simulink model "ALU1bit"  (R2024a)
settings: Solver=VariableStepAuto  StartTime=0.0  StopTime=10.0  RelTol=1e-3
settings Model: Creator=tusha  LastModifiedBy=tusha

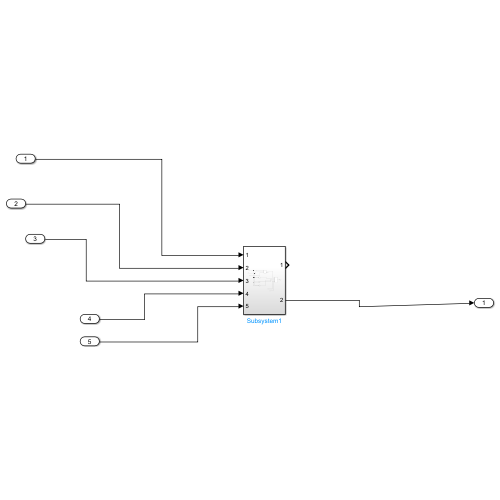
[thumbnail: Simulink's stored preview of the top-level diagram]
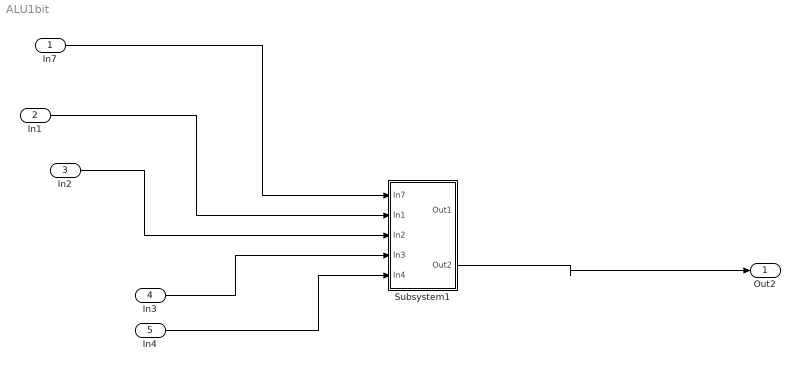
== system ALU1bit ==
  In7 : Inport
  In1 : Inport  Port=2
  In2 : Inport  Port=3
  In3 : Inport  Port=4
  In4 : Inport  Port=5
  Subsystem1 : Subsystem
  Out2 : Outport
  wires:
  In7/1 -> Subsystem1/1(In7)
  In1/1 -> Subsystem1/2(In1)
  In2/1 -> Subsystem1/3(In2)
  In3/1 -> Subsystem1/4(In3)
  In4/1 -> Subsystem1/5(In4)
  Subsystem1/2(Out2) -> Out2/1

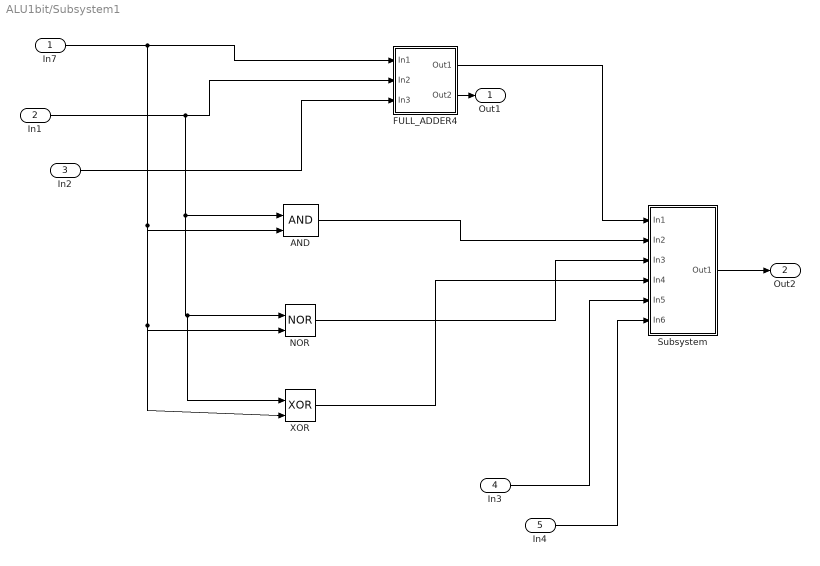
== system ALU1bit/Subsystem1 ==
  In7 : Inport
  In1 : Inport  Port=2
  In2 : Inport  Port=3
  In3 : Inport  Port=4
  In4 : Inport  Port=5
  AND : Logic  IconShape=distinctive  AllPortsSameDT=off  OutDataTypeStr=boolean
  FULL_ADDER4 : Subsystem
  NOR : Logic  Operator=NOR  IconShape=distinctive  AllPortsSameDT=off  OutDataTypeStr=boolean
  Subsystem : Subsystem
  XOR : Logic  Operator=XOR  IconShape=distinctive  AllPortsSameDT=off  OutDataTypeStr=boolean
  Out1 : Outport
  Out2 : Outport  Port=2
  wires:
  In7/1 -> XOR/2, NOR/2, AND/2, FULL_ADDER4/1(In1)
  Subsystem/1(Out1) -> Out2/1
  FULL_ADDER4/1(Out1) -> Subsystem/1(In1)
  In4/1 -> Subsystem/6(In6)
  In1/1 -> XOR/1, NOR/1, AND/1, FULL_ADDER4/2(In2)
  In2/1 -> FULL_ADDER4/3(In3)
  XOR/1 -> Subsystem/4(In4)
  AND/1 -> Subsystem/2(In2)
  NOR/1 -> Subsystem/3(In3)
  In3/1 -> Subsystem/5(In5)
  FULL_ADDER4/2(Out2) -> Out1/1

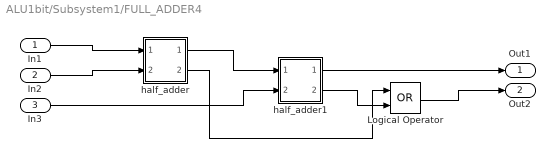
== system ALU1bit/Subsystem1/FULL_ADDER4 ==
  In1 : Inport
  In2 : Inport  Port=2
  In3 : Inport  Port=3
  Logical Operator : Logic  Operator=OR  AllPortsSameDT=off  OutDataTypeStr=boolean
  half_adder : Subsystem
  half_adder1 : Subsystem
  Out1 : Outport
  Out2 : Outport  Port=2
  wires:
  half_adder1/2(Out2) -> Logical Operator/2
  In3/1 -> half_adder1/2(In2)
  In1/1 -> half_adder/1(In1)
  half_adder1/1(Out1) -> Out1/1
  half_adder/1(Out1) -> half_adder1/1(In1)
  half_adder/2(Out2) -> Logical Operator/1
  In2/1 -> half_adder/2(In2)
  Logical Operator/1 -> Out2/1

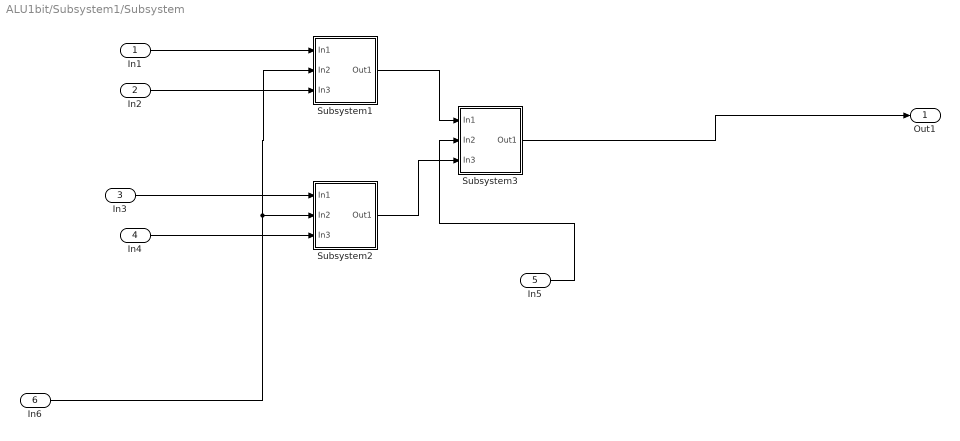
== system ALU1bit/Subsystem1/Subsystem ==
  In1 : Inport
  In2 : Inport  Port=2
  In3 : Inport  Port=3
  In4 : Inport  Port=4
  In5 : Inport  Port=5
  In6 : Inport  Port=6
  Subsystem1 : Subsystem
  Subsystem2 : Subsystem
  Subsystem3 : Subsystem
  Out1 : Outport
  wires:
  In6/1 -> Subsystem1/2(In2), Subsystem2/2(In2)
  In2/1 -> Subsystem1/3(In3)
  In3/1 -> Subsystem2/1(In1)
  Subsystem2/1(Out1) -> Subsystem3/3(In3)
  Subsystem1/1(Out1) -> Subsystem3/1(In1)
  In4/1 -> Subsystem2/3(In3)
  In1/1 -> Subsystem1/1(In1)
  In5/1 -> Subsystem3/2(In2)
  Subsystem3/1(Out1) -> Out1/1

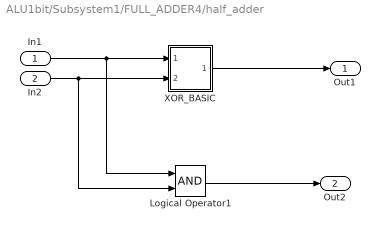
== system ALU1bit/Subsystem1/FULL_ADDER4/half_adder ==
  In1 : Inport
  In2 : Inport  Port=2
  Logical Operator1 : Logic  AllPortsSameDT=off  OutDataTypeStr=boolean
  XOR_BASIC : Subsystem
  Out1 : Outport
  Out2 : Outport  Port=2
  wires:
  In1/1 -> XOR_BASIC/1(In1), Logical Operator1/1
  In2/1 -> XOR_BASIC/2(In2), Logical Operator1/2
  Logical Operator1/1 -> Out2/1
  XOR_BASIC/1(Out1) -> Out1/1

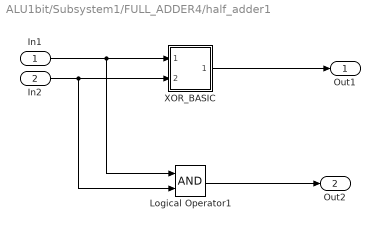
== system ALU1bit/Subsystem1/FULL_ADDER4/half_adder1 ==
  In1 : Inport
  In2 : Inport  Port=2
  Logical Operator1 : Logic  AllPortsSameDT=off  OutDataTypeStr=boolean
  XOR_BASIC : Subsystem
  Out1 : Outport
  Out2 : Outport  Port=2
  wires:
  In1/1 -> XOR_BASIC/1(In1), Logical Operator1/1
  In2/1 -> XOR_BASIC/2(In2), Logical Operator1/2
  Logical Operator1/1 -> Out2/1
  XOR_BASIC/1(Out1) -> Out1/1

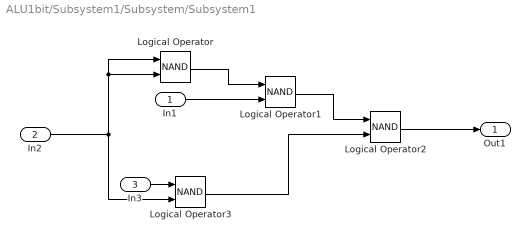
== system ALU1bit/Subsystem1/Subsystem/Subsystem1 ==
  In1 : Inport
  In2 : Inport  Port=2
  In3 : Inport  Port=3
  Logical Operator{,1..3} (4 alike) : Logic  Operator=NAND  AllPortsSameDT=off  OutDataTypeStr=boolean
  Out1 : Outport
  wires:
  Logical Operator2/1 -> Out1/1
  Logical Operator/1 -> Logical Operator1/1
  In2/1 -> Logical Operator/2, Logical Operator/1, Logical Operator3/2
  Logical Operator1/1 -> Logical Operator2/1
  In1/1 -> Logical Operator1/2
  Logical Operator3/1 -> Logical Operator2/2
  In3/1 -> Logical Operator3/1

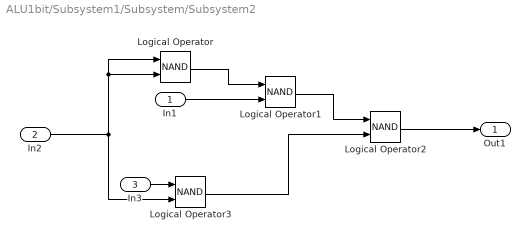
== system ALU1bit/Subsystem1/Subsystem/Subsystem2 ==
  In1 : Inport
  In2 : Inport  Port=2
  In3 : Inport  Port=3
  Logical Operator{,1..3} (4 alike) : Logic  Operator=NAND  AllPortsSameDT=off  OutDataTypeStr=boolean
  Out1 : Outport
  wires:
  Logical Operator2/1 -> Out1/1
  Logical Operator/1 -> Logical Operator1/1
  In2/1 -> Logical Operator/2, Logical Operator/1, Logical Operator3/2
  Logical Operator1/1 -> Logical Operator2/1
  In1/1 -> Logical Operator1/2
  Logical Operator3/1 -> Logical Operator2/2
  In3/1 -> Logical Operator3/1

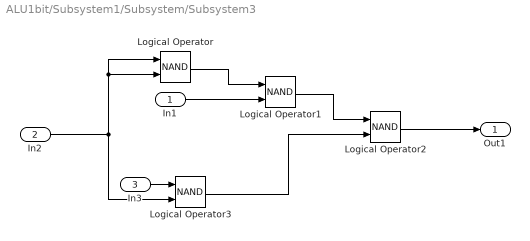
== system ALU1bit/Subsystem1/Subsystem/Subsystem3 ==
  In1 : Inport
  In2 : Inport  Port=2
  In3 : Inport  Port=3
  Logical Operator{,1..3} (4 alike) : Logic  Operator=NAND  AllPortsSameDT=off  OutDataTypeStr=boolean
  Out1 : Outport
  wires:
  Logical Operator2/1 -> Out1/1
  Logical Operator/1 -> Logical Operator1/1
  In2/1 -> Logical Operator/2, Logical Operator/1, Logical Operator3/2
  Logical Operator1/1 -> Logical Operator2/1
  In1/1 -> Logical Operator1/2
  Logical Operator3/1 -> Logical Operator2/2
  In3/1 -> Logical Operator3/1

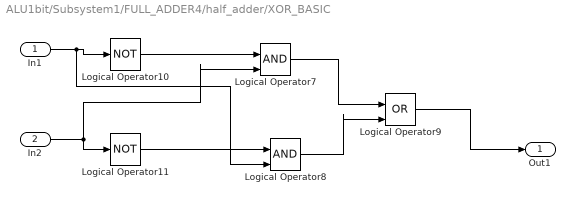
== system ALU1bit/Subsystem1/FULL_ADDER4/half_adder/XOR_BASIC ==
  In1 : Inport
  In2 : Inport  Port=2
  Logical Operator10 : Logic  Operator=NOT  IconShape=distinctive  AllPortsSameDT=off  OutDataTypeStr=boolean
  Logical Operator11 : Logic  Operator=NOT  IconShape=distinctive  AllPortsSameDT=off  OutDataTypeStr=boolean
  Logical Operator7 : Logic  IconShape=distinctive  AllPortsSameDT=off  OutDataTypeStr=boolean
  Logical Operator8 : Logic  IconShape=distinctive  AllPortsSameDT=off  OutDataTypeStr=boolean
  Logical Operator9 : Logic  Operator=OR  IconShape=distinctive  AllPortsSameDT=off  OutDataTypeStr=boolean
  Out1 : Outport
  wires:
  Logical Operator8/1 -> Logical Operator9/2
  Logical Operator7/1 -> Logical Operator9/1
  In2/1 -> Logical Operator7/2, Logical Operator11/1
  Logical Operator11/1 -> Logical Operator8/1
  Logical Operator9/1 -> Out1/1
  In1/1 -> Logical Operator8/2, Logical Operator10/1
  Logical Operator10/1 -> Logical Operator7/1

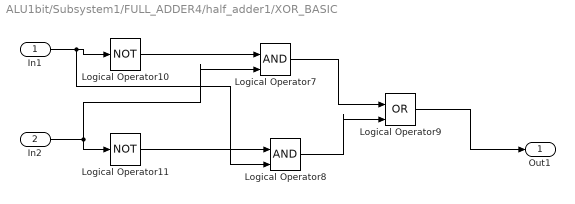
== system ALU1bit/Subsystem1/FULL_ADDER4/half_adder1/XOR_BASIC ==
  In1 : Inport
  In2 : Inport  Port=2
  Logical Operator10 : Logic  Operator=NOT  IconShape=distinctive  AllPortsSameDT=off  OutDataTypeStr=boolean
  Logical Operator11 : Logic  Operator=NOT  IconShape=distinctive  AllPortsSameDT=off  OutDataTypeStr=boolean
  Logical Operator7 : Logic  IconShape=distinctive  AllPortsSameDT=off  OutDataTypeStr=boolean
  Logical Operator8 : Logic  IconShape=distinctive  AllPortsSameDT=off  OutDataTypeStr=boolean
  Logical Operator9 : Logic  Operator=OR  IconShape=distinctive  AllPortsSameDT=off  OutDataTypeStr=boolean
  Out1 : Outport
  wires:
  Logical Operator8/1 -> Logical Operator9/2
  Logical Operator7/1 -> Logical Operator9/1
  In2/1 -> Logical Operator7/2, Logical Operator11/1
  Logical Operator11/1 -> Logical Operator8/1
  Logical Operator9/1 -> Out1/1
  In1/1 -> Logical Operator8/2, Logical Operator10/1
  Logical Operator10/1 -> Logical Operator7/1
